simulink model "close_noise"  (R2017a)
settings: Solver=VariableStepAuto  StartTime=0.0  StopTime=10.0  RelTol=1e-3
values from neighbouring files (symbols this model uses):
  Fs = 100    [TE_dg.m]    (also in close_loop_step_dg.m; close_loop_tf2_dg.m = 1000; multi_sin_damp_dg.m = 1000; open_loop_step_dg.m)
  noise_amplitude = 1e-5    (= 1e-05)    [multi_sin_damp_dg.m]    (also in open_noise_dg.m = 1; sin_damp_dg.m)
  seed = randi([0 1000],1)    [close_loop_step_dg.m]    (also in close_loop_tf2_dg.m; multi_sin_damp_dg.m; open_loop_step_dg.m; open_noise_dg.m)
  tau = 50    [testbench.m]
libraries: simulink x1
settings Model: Creator=ljxia  LastModifiedBy=ljxia

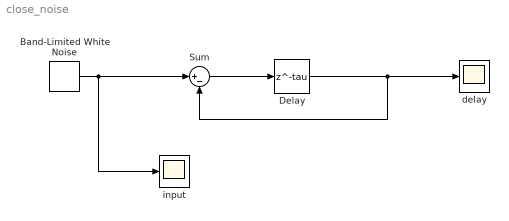
== system close_noise ==
  Band-Limited White Noise : simulink/Sources/Band-Limited White Noise  Cov=[noise_amplitude]  Ts=1/Fs  seed=[seed]
  Delay : Delay  DelayLength=tau  InitialCondition=0  SampleTime=1/Fs
  Sum : Sum  Inputs=|+-
  delay : Scope
  input : Scope
  wires:
  Delay/1 -> Sum/2, delay/1
  Band-Limited White Noise/1 -> Sum/1, input/1
  Sum/1 -> Delay/1
